simulink model "MSD"  (R2013a)
settings: Solver=ode45  StartTime=0.0  StopTime=5  RelTol=1e-3
settings Model: Creator=Ahmed  LastModifiedBy=Ahmed

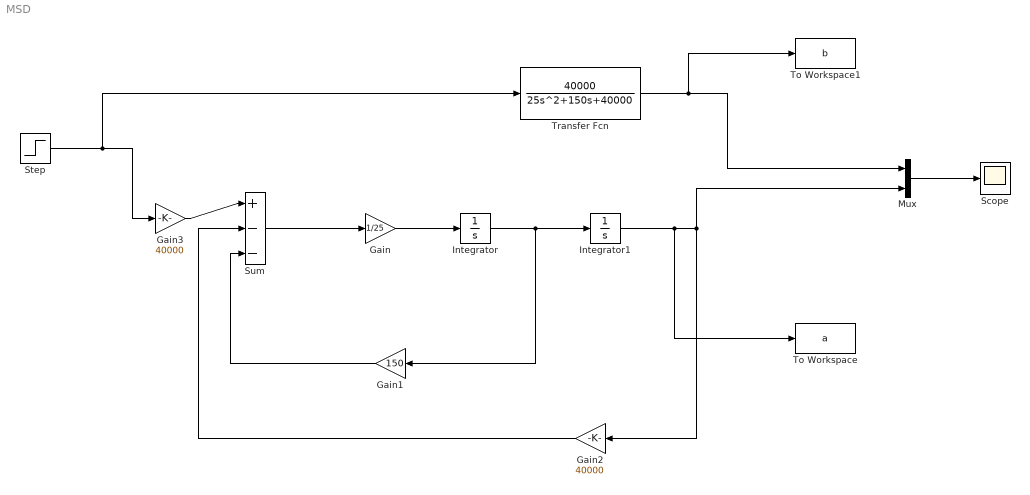
== system MSD ==
  Gain : Gain  Gain=1/25
  Gain1 : Gain  Gain=150
  Gain2 : Gain  Gain=40000
  Gain3 : Gain  Gain=40000
  Integrator : Integrator
  Integrator1 : Integrator
  Mux : Mux  Inputs=2
  Scope : Scope
  Step : Step  SampleTime=0
  Sum : Sum  Inputs=|+--
  To Workspace : ToWorkspace  VariableName=a  SampleTime=-1  SaveFormat=Timeseries
  To Workspace1 : ToWorkspace  VariableName=b  SampleTime=-1  SaveFormat=Timeseries
  Transfer Fcn : TransferFcn  Numerator=[40000]  Denominator=[25 150 40000]
  wires:
  Integrator/1 -> Gain1/1, Integrator1/1
  Gain/1 -> Integrator/1
  Sum/1 -> Gain/1
  Integrator1/1 -> To Workspace/1, Mux/2, Gain2/1
  Gain1/1 -> Sum/3
  Gain2/1 -> Sum/2
  Gain3/1 -> Sum/1
  Step/1 -> Transfer Fcn/1, Gain3/1
  Transfer Fcn/1 -> To Workspace1/1, Mux/1
  Mux/1 -> Scope/1
